simulink model "continuousPID_2018a"  (Simulink 9.1)
settings: Solver=ode45  StartTime=0.0  StopTime=10.0  MaxStep=.2  RelTol=1e-3  EnableMultiTasking=on
model workspace (MAT data in the model file):
  PID_TRESH : num (value not decoded)
undefined symbols (not defined in the file): DiscIntNeverNeededParam
libraries: simulink x1
settings Model: Creator=The MathWorks, Inc.  LastModifiedBy=gaoqiang
settings DataIOCC: LimitDataPoints=on
settings OptimizationCC: ExpressionDepthLimit=2147483647
settings DebuggingCC: SolverPrmCheckMsg=warning  FcnCallInpInsideContextMsg=warning  StateNameClashWarn=warning
settings SFSimCC: SimParseCustomCode=off
settings ConfigComp: CovHtmlReporting=off  CovSFcnEnable=off

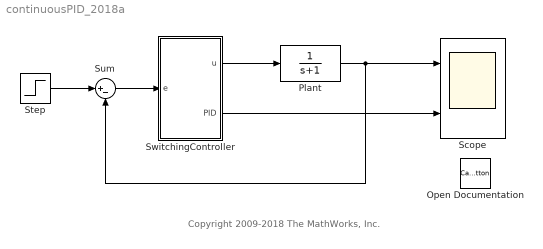
== system continuousPID_2018a ==
  note: Copyright 2009-2018 The MathWorks, Inc.
  Open Documentation : CallbackButton  WebBlockId=7  ButtonText=?
      settings: ClickFcn=showExample('stateflow/UsingSimulinkFunctionsToDesignSwitchingControllersExample')
  Plant : TransferFcn  Denominator=[1 1]
  Scope : Scope  NumInputPorts=2
  Step : Step  SampleTime=0
  Sum : Sum  Inputs=|+-
  SwitchingController : Stateflow chart  TreatAsAtomicUnit=on
  wires:
  Sum/1 -> SwitchingController/1(e)
  Plant/1 -> Sum/2, Scope/1
  SwitchingController/1(u) -> Plant/1
  Step/1 -> Sum/1
  SwitchingController/2(" PID") -> Scope/2

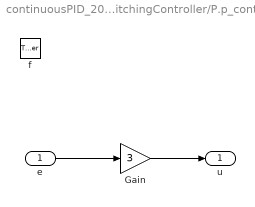
== system continuousPID_2018a/SwitchingController/P.p_control ==
  e : Inport
  f : TriggerPort  TriggerType=function-call  VariantControl=(inherit)
      settings: CopyFcn=Stateflow.SLINSF.SimulinkMan.removeBlockPreDeleteFcn  PreDeleteFcn=Stateflow.SLINSF.SimulinkMan.unsafePredeleteFcn
  Gain : Gain  Gain=3
  u : Outport
  wires:
  e/1 -> Gain/1
  Gain/1 -> u/1

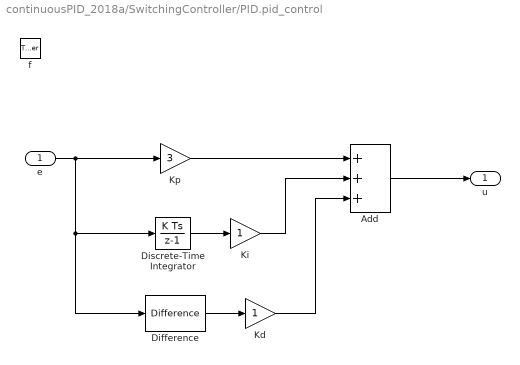
== system continuousPID_2018a/SwitchingController/PID.pid_control ==
  e : Inport
  f : TriggerPort  TriggerType=function-call  VariantControl=(inherit)
      settings: CopyFcn=Stateflow.SLINSF.SimulinkMan.removeBlockPreDeleteFcn  PreDeleteFcn=Stateflow.SLINSF.SimulinkMan.unsafePredeleteFcn
  Add : Sum  Inputs=+++
  Difference : simulink/Discrete/Difference  ICPrevInput=0.0  OutMin=[]  OutMax=[]  OutDataType=fixdt(1, 16)  OutScaling=2^-10  DoSatur=off
  Discrete-Time Integrator : DiscreteIntegrator  SampleTime=-1  ICPrevOutput=DiscIntNeverNeededParam  ICPrevScaledInput=DiscIntNeverNeededParam
  Kd : Gain
  Ki : Gain
  Kp : Gain  Gain=3
  u : Outport
  wires:
  e/1 -> Kp/1, Discrete-Time Integrator/1, Difference/1
  Kp/1 -> Add/1
  Add/1 -> u/1
  Discrete-Time Integrator/1 -> Ki/1
  Difference/1 -> Kd/1
  Ki/1 -> Add/2
  Kd/1 -> Add/3

== stateflow chart SwitchingController ==
  state STEADY
    entry: u = 0;
  state P
    du:
    u = p_control(e);
    state u = p_control(e) [function]
  state PID
    du:
    u = pid_control(e);
    state u = pid_control(e) [function]
  (default) -> STEADY
  P -> PID : [e < PID_TRESH]
  STEADY -> P : [e > 0.01]
  data: e function_input double; u function_output double; e function_input double; u function_output double; e input double; u output double; PID output boolean; PID_TRESH parameter double
